simulink model "ani12019a"  (R2021b)
settings: Solver=ode1  StartTime=0.0  StopTime=100  FixedStep=ts  RelTol=1e-3
values from neighbouring files (symbols this model uses):
  levitador = imrotate(levitador,90,'bilinear')    [Render.m]
  pelota = imrotate(pelota,90,'bilinear')    [Render.m]
  ts = 0.06    [Render.m]
  ventilador1 = imresize(ventilador1, scale)    [Render.m]
  ventilador2 = imresize(ventilador2, scale)    [Render.m]
libraries: androiduilib x4, cstblocks x1, slpidlib x1, androidaudiovideolib x1
settings Model: Creator=lberm  LastModifiedBy=hadr9
settings SolverCC: AlgebraicLoopSolver=TrustRegion
settings OptimizationCC: EnhancedBackFolding=on  PassReuseOutputArgsThreshold=0  MaxStackSize=64  OptimizeBlockOrder=speed  DifferentSizesBufferReuse=on  OptimizationCustomize=off
settings DebuggingCC: ParameterTunabilityLossMsg=error
settings HardwareCC: ProdBitPerPointer=32  ProdBitPerSizeT=32  ProdBitPerPtrDiffT=32  ProdLargestAtomicInteger=Long  ProdLargestAtomicFloat=Double  ProdWordSize=32  ProdHWDeviceType=ARM Compatible->ARM Cortex  UseEmbeddedCoderFeatures=off  UseSimulinkCoderFeatures=off
settings SFSimCC: MATLABDynamicMemAlloc=off  CustomCodeUndefinedFunction=UseInterfaceOnly
settings RTWCC: Description=Embedded Coder  SystemTargetFile=ert.tlc  HardwareBoard=Android Device  TLCOptions="-aInlineSetEventsForThisBaseRateFcn=TLC_FALSE -aSuppressMultiTaskScheduler=TLC_FALSE  -aRateBasedStepFcn=0"  TemplateMakefile=ert_default_tmf  RTWVerbose=off  Toolchain=Android SDK/NDK Tools
settings CodeAppCC: ForceParamTrailComments=on  OperatorAnnotations=on
settings ERTTargetCC: ERTCustomFileBanners=off  SupportContinuousTime=on  SupportNonInlinedSFcns=on  RemoveResetFunc=off  SupportVariableSizeSignals=on  ModelStepFunctionPrototypeControlCompliant=off

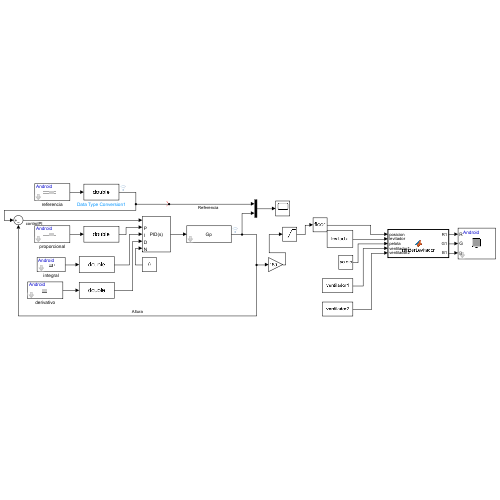
[thumbnail: Simulink's stored preview of the top-level diagram]
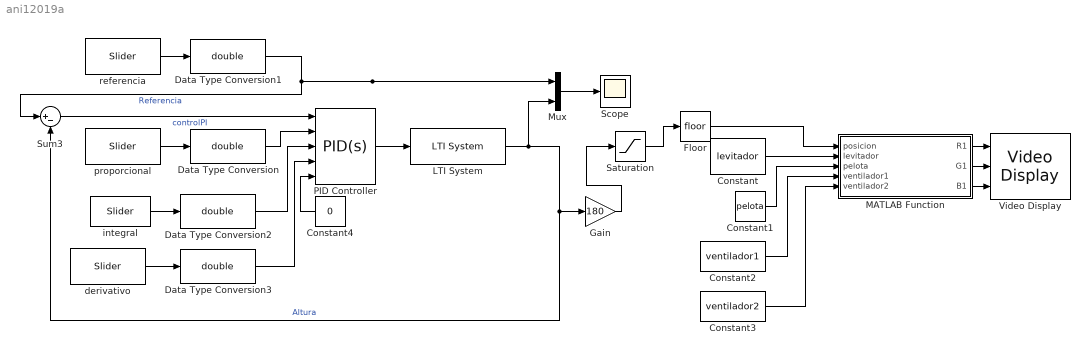
== system ani12019a ==
  Constant : Constant  Value=levitador  SampleTime=ts
  Constant1 : Constant  Value=pelota  SampleTime=ts
  Constant2 : Constant  Value=ventilador1  SampleTime=ts
  Constant3 : Constant  Value=ventilador2  SampleTime=ts
  Constant4 : Constant  Value=0
  Data Type Conversion{,1..3} (4 alike) : DataTypeConversion  OutDataTypeStr=double
  Floor : Rounding
  Gain : Gain  Gain=180
  LTI System : cstblocks/LTI System  sys=Gp  IC=[]
  MATLAB Function : MATLAB Function  TreatAsAtomicUnit=on
  Mux : Mux  Inputs=2
  PID Controller : slpidlib/PID Controller  Controller=PID  Form=Parallel  TimeDomain=Continuous-time  UseExternalTs=off  SampleTime=-1  IntegratorMethod=Forward Euler  FilterMethod=Forward Euler  ControllerParametersSource=external  P=1  I=1  D=1  UseFilter=on  N=100  TunerSelectOption=Transfer Function Based (PID Tuner App)  InitialConditionSource=internal  InitialConditionForIntegrator=0  InitialConditionForFilter=0  DifferentiatorICPrevScaledInput=0  ExternalReset=none  TrackingMode=off  Kt=1  LimitOutput=off  SatLimitsSource=internal  UpperSaturationLimit=inf  LowerSaturationLimit=-inf  LinearizeAsGain=on  AntiWindupMode=none  Kb=1  POutMin=[]  POutMax=[]  IOutMin=[]  IOutMax=[]  DOutMin=[]  DOutMax=[]  NOutMin=[]  NOutMax=[]  SumOutMin=[]  SumOutMax=[]  SaturationOutMin=[]  SaturationOutMax=[]  PParamMin=[]  PParamMax=[]  IParamMin=[]  IParamMax=[]  DParamMin=[]  DParamMax=[]  NParamMin=[]  NParamMax=[]  KbParamMin=[]  KbParamMax=[]  KtParamMin=[]  KtParamMax=[]  KbOutMin=[]  KbOutMax=[]  KtOutMin=[]  KtOutMax=[]  IntegratorOutMin=[]  IntegratorOutMax=[]  FilterOutMin=[]  FilterOutMax=[]  SumI1OutMin=[]  SumI1OutMax=[]  SumI2OutMin=[]  SumI2OutMax=[]  SumI3OutMin=[]  SumI3OutMax=[]  SumI4OutMin=[]  SumI4OutMax=[]  SumDOutMin=[]  SumDOutMax=[]  DifferentiatorOutMin=[]  DifferentiatorOutMax=[]  FilterDiffOutCoefMin=[]  FilterDiffOutCoefMax=[]  ReciprocalOutMin=[]  ReciprocalOutMax=[]  SumDenOutMin=[]  SumDenOutMax=[]  SumNumOutMin=[]  SumNumOutMax=[]  DivideOutMin=[]  DivideOutMax=[]  UdiffTsProdOutMin=[]  UdiffTsProdOutMax=[]  NTsProdOutMin=[]  NTsProdOutMax=[]  UintegralTsProdOutMin=[]  UintegralTsProdOutMax=[]  UngainTsProdOutMin=[]  UngainTsProdOutMax=[]  IntegratorContinuousStateAttributes=''  IntegratorStateMustResolveToSignalObject=off  IntegratorRTWStateStorageClass=Auto  FilterContinuousStateAttributes=''  FilterStateMustResolveToSignalObject=off  FilterRTWStateStorageClass=Auto  ParallelPVariant=ExternalParameters  IdealPVariant=Disabled  IVariant=ExternalParameters  DVariant=ExternalParameters  IntegratorVariant=Continuous  SatVariant=Disabled  AWVariant=Passthrough  PCopyVariant=Disabled  TRVariant=Disabled  FdbkBlocksVariant=Forward  IdealPFdbkVariant=Disabled  SatFdbkVariant=Disabled  DerivativeFilterVariant=ContFilter  NVariant=ExternalParameters  NCopyVariant=Disabled  FilterICVariant=InternalICsFilter  IntegratorICVariant=InternalICs  ExternalResetVariant=Disabled  TRSumVariant=Passthrough  SumFdbkVariant=Disabled  SumVariant=Sum_PID  TsampFilterVariant=InternalTs  TsampNgainVariant=Passthrough  TsampIntegralVariant=Passthrough  ExternalSaturationOutDataTypeStr=Inherit: Same as second input
  Saturation : Saturate  UpperLimit=180  LowerLimit=0
  Scope : Scope
  Sum3 : Sum  Inputs=|+-  OutDataTypeStr=double
  Video Display : androidaudiovideolib/Video Display  BlockPlatform=Android
      settings: SourceProductBaseCode=ANDROID
  derivativo : androiduilib/Slider  Min=1  Value=1  Max=10  Resolution=0.01  SliderId=ani12019a/derivativo  SampleTime=ts  BlockPlatform=Android
      settings: SourceProductBaseCode=ANDROID
  integral : androiduilib/Slider  Min=1  Value=1  Max=10  Resolution=0.1  SliderId=ani12019a/integral  SampleTime=ts  BlockPlatform=Android
      settings: SourceProductBaseCode=ANDROID
  proporcional : androiduilib/Slider  Min=1  Value=1  Max=10  Resolution=0.01  SliderId=ani12019a/proporcional  SampleTime=ts  BlockPlatform=Android
      settings: SourceProductBaseCode=ANDROID
  referencia : androiduilib/Slider  Min=0.01  Value=0.5  Max=1  Resolution=0.01  SliderId=ani12019a/referencia  SampleTime=ts  BlockPlatform=Android
      settings: SourceProductBaseCode=ANDROID
  wires:
  Saturation/1 -> Floor/1
  Mux/1 -> Scope/1
  Gain/1 -> Saturation/1
  proporcional/1 -> Data Type Conversion/1
  Data Type Conversion1/1 -> Sum3/1, Mux/1  "Referencia"
  referencia/1 -> Data Type Conversion1/1
  integral/1 -> Data Type Conversion2/1
  MATLAB Function/1(R1) -> Video Display/1
  MATLAB Function/2(G1) -> Video Display/2
  MATLAB Function/3(B1) -> Video Display/3
  Floor/1 -> MATLAB Function/1(posicion)
  Constant/1 -> MATLAB Function/2(levitador)
  Constant1/1 -> MATLAB Function/3(pelota)
  Constant2/1 -> MATLAB Function/4(ventilador1)
  Constant3/1 -> MATLAB Function/5(ventilador2)
  PID Controller/1 -> LTI System/1
  derivativo/1 -> Data Type Conversion3/1
  Sum3/1 -> PID Controller/1  "controlPI"
  Data Type Conversion/1 -> PID Controller/2
  Data Type Conversion2/1 -> PID Controller/3
  Data Type Conversion3/1 -> PID Controller/4
  LTI System/1 -> Gain/1, Sum3/2, Mux/2  "Altura"
  Constant4/1 -> PID Controller/5

== matlab function ani12019a/MATLAB Function ==
  data: posicion input; R1 output; G1 output; B1 output; levitador input; pelota input; ventilador1 input; ventilador2 input
function [R1,G1,B1] = renderLevitador(posicion,levitador,pelota,ventilador1,ventilador2)

if mod((posicion),2)==1
    ventilador=ventilador1;
else
    ventilador=ventilador2;
end

r=ventilador(:,:,1);
g=ventilador(:,:,2);
b=ventilador(:,:,3);
x=220;
y=426;

[n,m]=size(r);
for i=1:n
    for j=1:m
        if r(i,j)<=250 &&  g(i,j)<=250 && b(i,j)<=250
          levitador(i+x,j+y,:)=ventilador(i,j,:);
        end
    end
end

r=pelota(:,:,1);
g=pelota(:,:,2);
b=pelota(:,:,3);

ymax=380;
x=208;

[n,m]=size(r);
for i=1:n
    for j=1:m
        if r(i,j)<=245 &&  g(i,j)<=245 && b(i,j)<=245
          levitador(i+x,j+ymax-posicion,:)=pelota(i,j,:);
        end
    end
end

R1 = uint8(zeros(480,640));
G1 = uint8(zeros(480,640));
B1 = uint8(zeros(480,640));

G1 = levitador(:,:,3);
B1 = levitador(:,:,2);
R1 = levitador(:,:,1);
